simulink model "oppg1"  (R2017a)
settings: Solver=VariableStepAuto  StartTime=0.0  StopTime=100  RelTol=1e-3
settings Model: Creator=siguhe  LastModifiedBy=siguhe

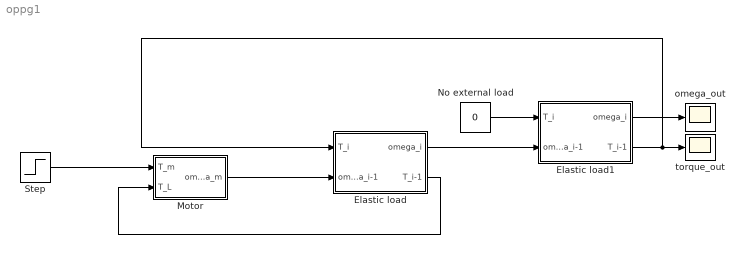
== system oppg1 ==
  Elastic load : Subsystem
  Elastic load1 : Subsystem
  Motor : Subsystem
  No external load : Constant  Value=0
  Step : Step  SampleTime=0
  omega_out : Scope
  torque_out : Scope
  wires:
  Elastic load/1(omega_i) -> Elastic load1/2(omega_i-1)
  Motor/1(omega_m) -> Elastic load/2(omega_i-1)
  Elastic load1/2(T_i-1) -> Elastic load/1(T_i), torque_out/1
  Step/1 -> Motor/1(T_m)
  Elastic load/2(T_i-1) -> Motor/2(T_L)
  No external load/1 -> Elastic load1/1(T_i)
  Elastic load1/1(omega_i) -> omega_out/1

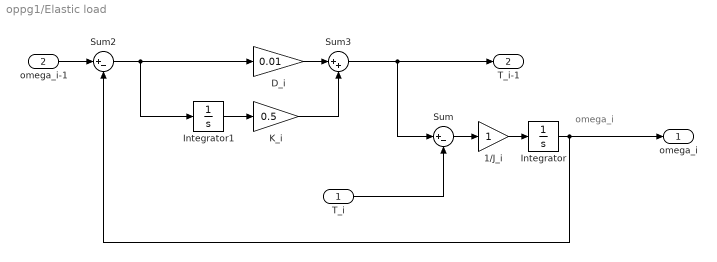
== system oppg1/Elastic load ==
  note: omega_i
  T_i : Inport
  omega_i-1 : Inport  Port=2
  1/J_i : Gain
  D_i : Gain  Gain=0.01
  Integrator : Integrator
  Integrator1 : Integrator
  K_i : Gain  Gain=0.5
  Sum : Sum  Inputs=|+-
  Sum2 : Sum  Inputs=|+-
  Sum3 : Sum  Inputs=|++
  omega_i : Outport
  T_i-1 : Outport  Port=2
  wires:
  1/J_i/1 -> Integrator/1
  Sum/1 -> 1/J_i/1
  Sum2/1 -> Integrator1/1, D_i/1
  K_i/1 -> Sum3/2
  D_i/1 -> Sum3/1
  Integrator/1 -> Sum2/2, omega_i/1
  T_i/1 -> Sum/2
  Sum3/1 -> Sum/1, T_i-1/1
  omega_i-1/1 -> Sum2/1
  Integrator1/1 -> K_i/1

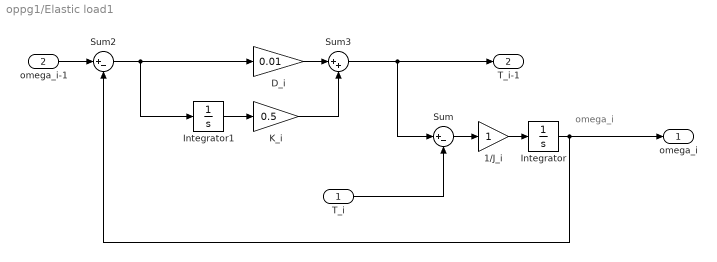
== system oppg1/Elastic load1 ==
  note: omega_i
  T_i : Inport
  omega_i-1 : Inport  Port=2
  1/J_i : Gain
  D_i : Gain  Gain=0.01
  Integrator : Integrator
  Integrator1 : Integrator
  K_i : Gain  Gain=0.5
  Sum : Sum  Inputs=|+-
  Sum2 : Sum  Inputs=|+-
  Sum3 : Sum  Inputs=|++
  omega_i : Outport
  T_i-1 : Outport  Port=2
  wires:
  1/J_i/1 -> Integrator/1
  Sum/1 -> 1/J_i/1
  Sum2/1 -> Integrator1/1, D_i/1
  K_i/1 -> Sum3/2
  D_i/1 -> Sum3/1
  Integrator/1 -> Sum2/2, omega_i/1
  T_i/1 -> Sum/2
  Sum3/1 -> Sum/1, T_i-1/1
  omega_i-1/1 -> Sum2/1
  Integrator1/1 -> K_i/1

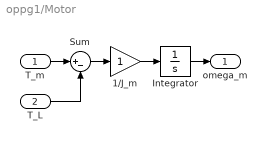
== system oppg1/Motor ==
  T_m : Inport
  T_L : Inport  Port=2
  "1/J_m " : Gain
  Integrator : Integrator
  Sum : Sum  Inputs=|+-
  omega_m : Outport
  wires:
  "1/J_m "/1 -> Integrator/1
  Sum/1 -> "1/J_m "/1
  T_L/1 -> Sum/2
  Integrator/1 -> omega_m/1
  T_m/1 -> Sum/1
